simulink model "PM"  (R2023b)
settings: Solver=FixedStepAuto  StartTime=0.0  StopTime=10  FixedStep=0.001  RelTol=1e-3
settings Model: Creator=HP  LastModifiedBy=HP

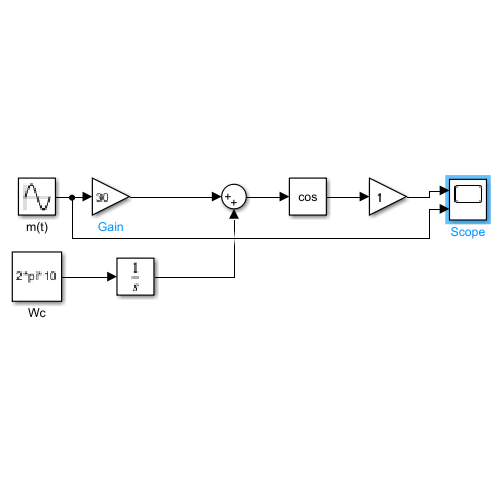
[thumbnail: Simulink's stored preview of the top-level diagram]
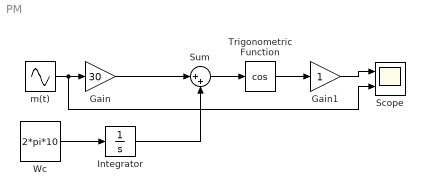
== system PM ==
  Gain : Gain  Gain=30
  Gain1 : Gain
  Integrator : Integrator
  Scope : Scope  NumInputPorts=2
  Sum : Sum  Inputs=|++
  Trigonometric Function : Trigonometry  Operator=cos
  Wc : Constant  Value=2*pi*10
  m(t) : Sin  Frequency=1*2*pi  SampleTime=0
  wires:
  m(t)/1 -> Scope/2, Gain/1
  Gain/1 -> Sum/1
  Wc/1 -> Integrator/1
  Integrator/1 -> Sum/2
  Sum/1 -> Trigonometric Function/1
  Trigonometric Function/1 -> Gain1/1
  Gain1/1 -> Scope/1
